simulink model "EchoAndReverberationDSKC6713"  (Simulink 6.5)
settings: Solver=FixedStepDiscrete  StartTime=0.0  StopTime=inf  RelTol=1e-3
undefined symbols (not defined in the file or in its folder): bit
libraries: simulink x6, c6713dsklib x3, c6000tgtpreflib x1
settings Model: Creator=Administrator  LastModifiedBy=Administrator  ProdHWDeviceType=TI C6000
settings SolverCC: PositivePriorityOrder=on
settings DataIOCC: SaveOutput=off  SaveTime=off
settings OptimizationCC: OptimizeModelRefInitCode=on
settings HardwareCC: ProdBitPerLong=40  ProdIntDivRoundTo=Zero  ProdEndianess=LittleEndian  ProdHWDeviceType=TI C6000
settings RTWCC: SystemTargetFile=ti_c6000_ert.tlc  GenCodeOnly=on  TemplateMakefile=ti_c6000_ert.tmf  Description=Embedded Target for TI C6000 DSP (ERT)  ProcessScript=ti_c6000_ert_make_rtw_hook
settings CodeAppCC: IgnoreCustomStorageClasses=off
settings C6000ERTTargetCC: TargetFcnLib=ansi_tfl_tmw.mat  GenFloatMathFcnCalls=ANSI_C  UtilityFuncGeneration=Auto  GenerateFullHeader=on  GenerateSampleERTMain=off  GenerateTestInterfaces=off  IsPILTarget=off  ModelReferenceCompliant=on  IncludeMdlTerminateFcn=on  CombineOutputUpdateFcns=on  SuppressErrorStatus=off  IncludeFileDelimiter=Auto  ERTCustomFileBanners=on  SupportAbsoluteTime=on  LogVarNameModifier=rt_  MatFileLogging=off  MultiInstanceERTCode=off  SupportNonFinite=on  SupportComplex=on  PurelyIntegerCode=off  SupportContinuousTime=off  SupportNonInlinedSFcns=off  EnableShiftOperators=on  ParenthesesLevel=Nominal  GenerateErtSFunction=off  GenerateASAP2=off  ExtMode=off  ExtModeTransport=0  ExtModeStaticAlloc=off  ExtModeStaticAllocSize=1000000  ExtModeTesting=off  ExtModeMexFile=ext_comm  InlinedParameterPlacement=NonHierarchical  TargetOS=BareBoardExample  MultiInstanceErrorCode=Error  RateGroupingCode=on  RootIOFormat=Individual arguments  RTWCAPISignals=off  RTWCAPIParams=off  RTWCAPIStates=off  ERTSrcFileBannerTemplate=ert_code_template.cgt  ERTHdrFileBannerTemplate=ert_code_template.cgt  ERTDataSrcFileTemplate=ert_code_template.cgt  ERTDataHdrFileTemplate=ert_code_template.cgt  ERTCustomFileTemplate=example_file_process.tlc  ModuleNamingRule=Unspecified  SignalDisplayLevel=10  ParamTuneLevel=10  GlobalDataDefinition=Auto  DataDefinitionFile=global.c  GlobalDataReference=Auto  DataReferenceFile=global.h  GRTInterface=off  EnableUserReplacementTypes=off  MemSecPackage=--- None ---  MemSecDataConstants=Default  MemSecDataIO=Default  MemSecDataInternal=Default  MemSecDataParameters=Default  MemSecFuncInitTerm=Default  MemSecFuncExecute=Default  exportCCSObj=on  ccsObjName=CCS_Obj  useDSPBIOS=on  ProfileGenCode=off  InlineDSPBlks=on  FPopt=off  memModel=Far_Aggregate  optLevel=Function(-o2)  CompilerVerbosity=Quiet  InterruptThreshOnC6x=off  SymbolicDebugOnC6x=off  RetainAsmFiles=off  RetainObjFiles=on  CreateMapFile=on  UserStackSize=8192  c6000BuildAction=Build_and_execute  OverrunAction=Notify_and_continue  OverrunNotificationMethod=Turn_on_LEDs

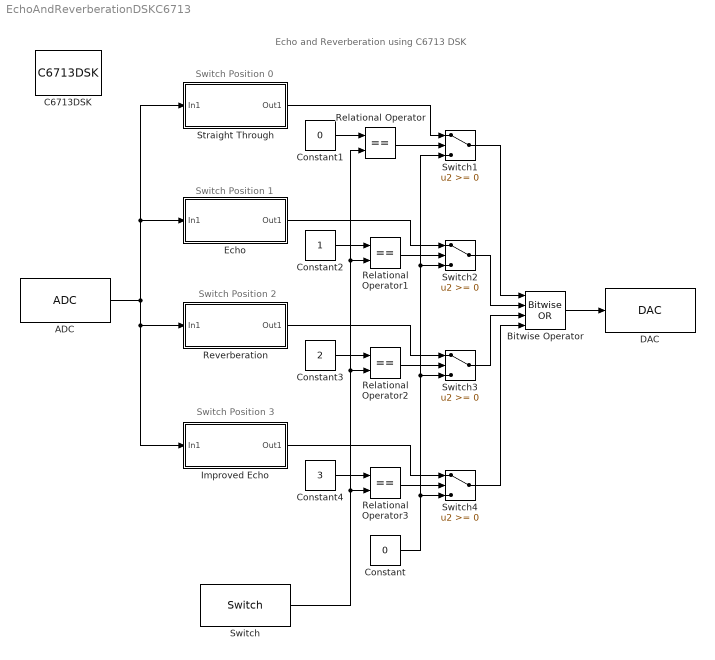
== system EchoAndReverberationDSKC6713 ==
  note: Echo and Reverberation using C6713 DSK
  note: Switch Position 0
  note: Switch Position 1
  note: Switch Position 2
  note: Switch Position 3
  ADC : c6713dsklib/ADC  ADCsource=Mic In  MicGain=on  Stereo=off  SampleRate=8 kHz  CodecDataFormat=16-bit  OutputDataType=Integer  Scaling=Normalize  SourceGain=0.0  FrameSize=1  inheritSampleTime=off
  Bitwise Operator : simulink/Logic and Bit Operations/Bitwise Operator  logicop=OR  UseBitMask=off  NumInputPorts=4  BitMask=bin2dec('11011001')  BitMaskRealWorld=Stored Integer
  C6713DSK : c6000tgtpreflib/C6713DSK  Tag=C6000 TARGET PREFERENCES BLOCK  SystemSampleTime=-1
  Constant : Constant  Value=0  OutDataTypeMode=int16  OutDataType=sfix(16)  ConRadixGroup=Use specified scaling  OutScaling=2^0  SampleTime=inf  FramePeriod=inf
  Constant1 : Constant  Value=0  OutDataTypeMode=int16  OutDataType=sfix(16)  ConRadixGroup=Use specified scaling  OutScaling=2^0  SampleTime=inf  FramePeriod=inf
  Constant2 : Constant  Value=1  OutDataTypeMode=int16  OutDataType=sfix(16)  ConRadixGroup=Use specified scaling  OutScaling=2^0  SampleTime=inf  FramePeriod=inf
  Constant3 : Constant  Value=2  OutDataTypeMode=int16  OutDataType=sfix(16)  ConRadixGroup=Use specified scaling  OutScaling=2^0  SampleTime=inf  FramePeriod=inf
  Constant4 : Constant  Value=3  OutDataTypeMode=int16  OutDataType=sfix(16)  ConRadixGroup=Use specified scaling  OutScaling=2^0  SampleTime=inf  FramePeriod=inf
  DAC : c6713dsklib/DAC  CodecDataFormat=16-bit  SampleRate=8 kHz  Scaling=Integer Value  DacAtten=0.0  OverflowMode=Saturate
  Echo : Subsystem
  Improved Echo : Subsystem
  Relational Operator{,1..3} (4 alike) : RelationalOperator  Operator===  LogicOutDataTypeMode=Boolean
  Reverberation : Subsystem
  Straight Through : Subsystem
  Switch : c6713dsklib/Switch  sw0=on  sw1=on  sw2=on  sw3=on  dType=Integer  Ts=-1
  Switch{1..4} (4 alike) : Switch
  wires:
  Bitwise Operator/1 -> DAC/1
  Relational Operator/1 -> Switch1/2
  Straight Through/1(Out1) -> Switch1/1
  Constant/1 -> Switch1/3, Switch2/3, Switch3/3, Switch4/3
  Switch1/1 -> Bitwise Operator/1
  Constant1/1 -> Relational Operator/1
  Switch/1 -> Relational Operator/2, Relational Operator1/2, Relational Operator2/2, Relational Operator3/2
  Switch2/1 -> Bitwise Operator/2
  Relational Operator1/1 -> Switch2/2
  Echo/1(Out1) -> Switch2/1
  Constant2/1 -> Relational Operator1/1
  Switch3/1 -> Bitwise Operator/3
  Relational Operator2/1 -> Switch3/2
  Constant3/1 -> Relational Operator2/1
  Reverberation/1(Out1) -> Switch3/1
  ADC/1 -> Straight Through/1(In1), Echo/1(In1), Reverberation/1(In1), Improved Echo/1(In1)
  Switch4/1 -> Bitwise Operator/4
  Relational Operator3/1 -> Switch4/2
  Improved Echo/1(Out1) -> Switch4/1
  Constant4/1 -> Relational Operator3/1

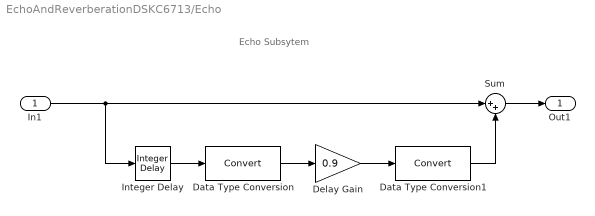
== system EchoAndReverberationDSKC6713/Echo ==
  note: Echo Subsytem
  In1 : Inport
  Data Type Conversion : DataTypeConversion  OutDataTypeMode=single
  Data Type Conversion1 : DataTypeConversion  OutDataTypeMode=int16
  Delay Gain : Gain  Gain=0.9
  Integer Delay : simulink/Discrete/Integer Delay  vinit=0  samptime=-1  NumDelays=4000
  Sum : Sum  Inputs=|++
  Out1 : Outport
  wires:
  In1/1 -> Integer Delay/1, Sum/1
  Integer Delay/1 -> Data Type Conversion/1
  Sum/1 -> Out1/1
  Data Type Conversion/1 -> Delay Gain/1
  Delay Gain/1 -> Data Type Conversion1/1
  Data Type Conversion1/1 -> Sum/2

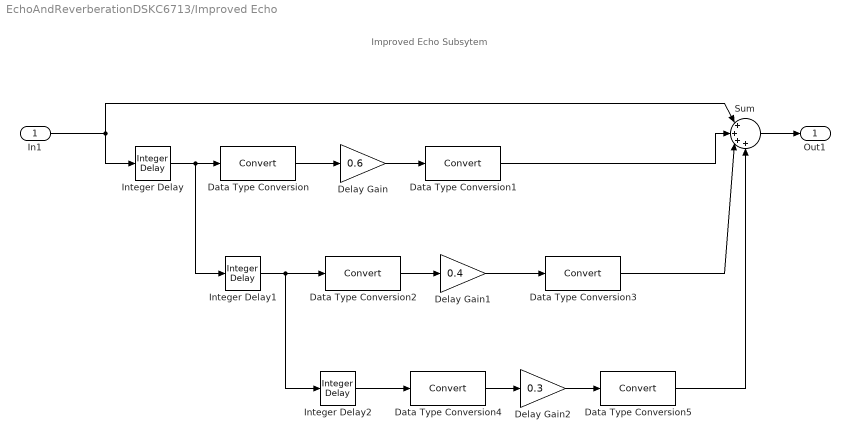
== system EchoAndReverberationDSKC6713/Improved Echo ==
  note: Improved Echo Subsytem
  In1 : Inport
  Data Type Conversion : DataTypeConversion  OutDataTypeMode=single
  Data Type Conversion1 : DataTypeConversion  OutDataTypeMode=int16
  Data Type Conversion2 : DataTypeConversion  OutDataTypeMode=single
  Data Type Conversion3 : DataTypeConversion  OutDataTypeMode=int16
  Data Type Conversion4 : DataTypeConversion  OutDataTypeMode=single
  Data Type Conversion5 : DataTypeConversion  OutDataTypeMode=int16
  Delay Gain : Gain  Gain=0.6
  Delay Gain1 : Gain  Gain=0.4
  Delay Gain2 : Gain  Gain=0.3
  Integer Delay : simulink/Discrete/Integer Delay  vinit=0  samptime=-1  NumDelays=1000
  Integer Delay1 : simulink/Discrete/Integer Delay  vinit=0  samptime=-1  NumDelays=1000
  Integer Delay2 : simulink/Discrete/Integer Delay  vinit=0  samptime=-1  NumDelays=1000
  Sum : Sum  Inputs=|++++
  Out1 : Outport
  wires:
  In1/1 -> Integer Delay/1, Sum/1
  Integer Delay/1 -> Data Type Conversion/1, Integer Delay1/1
  Sum/1 -> Out1/1
  Data Type Conversion/1 -> Delay Gain/1
  Delay Gain/1 -> Data Type Conversion1/1
  Data Type Conversion1/1 -> Sum/2
  Delay Gain1/1 -> Data Type Conversion3/1
  Data Type Conversion2/1 -> Delay Gain1/1
  Integer Delay1/1 -> Data Type Conversion2/1, Integer Delay2/1
  Data Type Conversion3/1 -> Sum/3
  Integer Delay2/1 -> Data Type Conversion4/1
  Data Type Conversion4/1 -> Delay Gain2/1
  Delay Gain2/1 -> Data Type Conversion5/1
  Data Type Conversion5/1 -> Sum/4

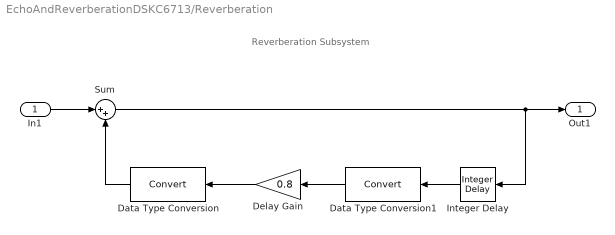
== system EchoAndReverberationDSKC6713/Reverberation ==
  note: Reverberation Subsystem
  In1 : Inport
  Data Type Conversion : DataTypeConversion  Orientation=left  OutDataTypeMode=int16
  Data Type Conversion1 : DataTypeConversion  Orientation=left  OutDataTypeMode=single
  Delay Gain : Gain  Orientation=left  Gain=0.8
  Integer Delay : simulink/Discrete/Integer Delay  Orientation=left  vinit=0  samptime=-1  NumDelays=800
  Sum : Sum  Inputs=|++
  Out1 : Outport
  wires:
  In1/1 -> Sum/1
  Sum/1 -> Out1/1, Integer Delay/1
  Integer Delay/1 -> Data Type Conversion1/1
  Data Type Conversion1/1 -> Delay Gain/1
  Delay Gain/1 -> Data Type Conversion/1
  Data Type Conversion/1 -> Sum/2

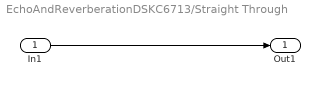
== system EchoAndReverberationDSKC6713/Straight Through ==
  In1 : Inport
  Out1 : Outport
  wires:
  In1/1 -> Out1/1
